simulink model "lab_4_equalizer_lms_buffer"  (R2012b)
settings: Solver=ode45  StartTime=0.0  StopTime=0.0012  RelTol=1e-3
values from neighbouring files (symbols this model uses):
  mu = 0.1    [lab_4_parameters.m]
  Ts = 1/Rs    (= 2.23214285714e-06)    [lab_4_parameters.m]
undefined symbols (not defined in the file or in its folder): dfilt, Fs, sided, Two
libraries: dspobslib x10, dspsigops x4, commsink2 x3, dspsnks4 x2, commchan3 x2, commdigbbndpm3 x2, dsparch4 x1, commrandsrc2 x1
settings Model: Creator=yuw  LastModifiedBy=yuw
settings OptimizationCC: InlineInvariantSignals=on  InitFltsAndDblsToZero=on
settings DebuggingCC: SaveWithParameterizedLinksMsg=none  SignalResolutionControl=TryResolveAllWithWarning  MultiTaskDSMMsg=warning  MultiTaskCondExecSysMsg=none  StrictBusMsg=None
settings RTWCC: IncludeERTFirstTime=on
settings GRTTargetCC: TargetFcnLib=ansi_tfl_tmw.mat  CombineOutputUpdateFcns=off  GRTInterface=on

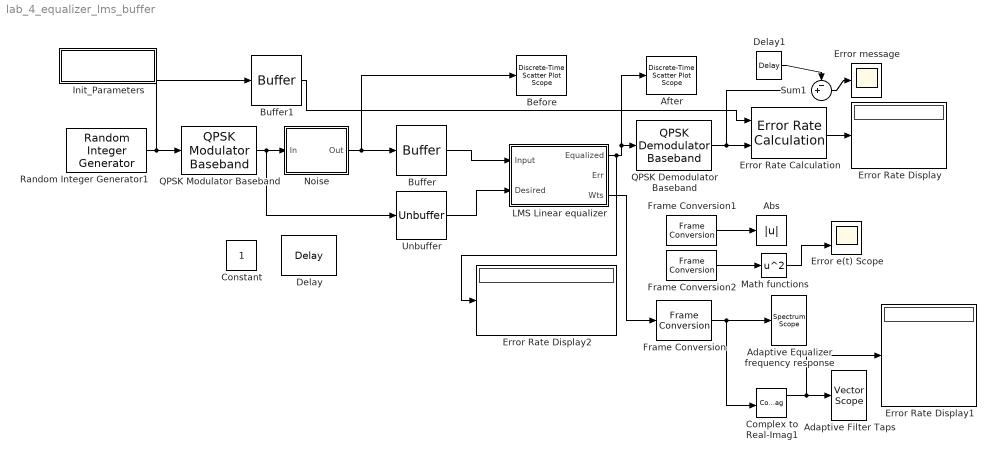
== system lab_4_equalizer_lms_buffer ==
  Abs : Abs
  Adaptive Equalizer frequency response : dspsnks4/Spectrum Scope  ScopeProperties=on  Domain=Frequency  HorizSpan=1  UseBuffer=off  BufferSize=128  Overlap=64  TreatMby1Signals=One channel  inpFftLenInherit=on  FFTlength=128  numAvg=2  DisplayProperties=off  AxisGrid=on  Memory=off  FrameNumber=on  AxisLegend=off  AxisZoom=off  OpenScopeAtSimStart=on  OpenScopeImmediately=off  FigPos=[8 424 450 170]  AxisProperties=off  XUnits=Hertz  XRange=Two-sided ((-Fs/2...Fs/2])  XDisplay=0  InheritXIncr=off  XIncr=1e-5  XLabel=Samples  XLimit=Auto  YUnits=dBW/Hertz  XMax=1  XMin=0  YLabel=Magnitude-squared, dB  LineProperties=off  LineStyles=--  LineMarkers=None  LineColors=[1 0 0]  wintypeSpecScope=Hann  RsSpecScope=50  betaSpecScope=5  winsampSpecScope=Periodic  XAxisParamsVer=6.8  isFrameUpgraded=on
      link override Periodogram: inheritFFT=off  inheritTs=off
      settings: YMin=-5.7892131592501  YMax=-3.17780882405879
  Adaptive Filter Taps : dspsnks4/Vector Scope  ScopeProperties=on  Domain=User-defined  HorizSpan=1  DisplayProperties=off  AxisGrid=on  Memory=off  FrameNumber=on  AxisLegend=off  AxisZoom=off  OpenScopeAtSimStart=on  OpenScopeImmediately=off  FigPos=[486 427 450 170]  AxisProperties=off  XUnits=Hertz  XRange=[0...Fs/2]  InheritXIncr=off  XIncr=1  XLabel=Coefficient Index  XLimit=Auto  XMin=0  XMax=1  XStart=0  YUnits=dB  YLabel=Amplitude  LineProperties=off  LineMarkers=.  XAxisParamsVer=6.8
      settings: YMin=-0.176505999051535  YMax=1.03663535601714
  After : commsink2/Discrete-Time Scatter Plot Scope  Tag=ScatterPlot  sampPerSymb=1  offsetEye=0  numTraces=400  numNewFrames=10  LineMarkers=.  LineColors=b  fading=on  render=on  AxisGrid=on  xMin=-1.5  xMax=1.5  yMin=-1.5  yMax=1.5  inphaseLabel=In-phase Amplitude  quadratureLabel=Quadrature Amplitude  openScopeAtSimStart=off  FrameNumber=off  FigPos=[420 374 400 400]  figTitle=Scatter Plot  numLinesMax=8  block_type_=scatter
  Before : commsink2/Discrete-Time Scatter Plot Scope  Tag=ScatterPlot  sampPerSymb=1  offsetEye=0  numTraces=400  numNewFrames=10  LineMarkers=.  LineColors=b  fading=on  render=on  AxisGrid=on  xMin=-1.5  xMax=1.5  yMin=-1.5  yMax=1.5  inphaseLabel=In-phase Amplitude  quadratureLabel=Quadrature Amplitude  openScopeAtSimStart=off  FrameNumber=off  FigPos=[10 374 400 400]  figTitle=Scatter Plot  numLinesMax=8  block_type_=scatter
  Buffer : Buffer  N=4
  Buffer1 : Buffer  N=10
  Complex to Real-Imag1 : ComplexToRealImag
  Constant : Constant
  Delay : dspsigops/Delay  InputProcessing=Inherited (this choice will be removed - see release notes)  dly_unit=Samples  delay=0  ic_detail=off  dif_ic_for_ch=off  dif_ic_for_dly=off  ic=0  reset_popup=None
  Delay1 : dspsigops/Delay  InputProcessing=Inherited (this choice will be removed - see release notes)  dly_unit=Samples  delay=4  ic_detail=off  dif_ic_for_ch=off  dif_ic_for_dly=off  ic=0  reset_popup=None
  Error Rate Calculation : commsink2/Error Rate Calculation  N=4  st_delay=0  cp_mode=Entire frame  subframe=[]  PMode=Port  WsName=ErrorVec  RsMode2=off  stop=off  numErr=100  maxBits=1e6
  Error Rate Display : Display
  Error Rate Display1 : Display
  Error Rate Display2 : Display
  Error e(t) Scope : Scope  NumInputPorts=2
      settings: TimeRange=1  YMin=5.55112e-017~-5  YMax=1.1~5  MaxDataPoints=10000
  Error message : Scope
      settings: TimeRange=1  YMin=-3  YMax=0  MaxDataPoints=10000
  Frame Conversion : FrameConversion
  Frame Conversion1 : FrameConversion  OutFrame=Sample-based
  Frame Conversion2 : FrameConversion  OutFrame=Sample-based
  Init_Parameters : Subsystem
      settings: OpenFcn=lab_4_parameters
      mask Display: disp('lab_4_parameters')
  LMS Linear equalizer : Subsystem
  Math functions : Math  Operator=square  SaturateOnIntegerOverflow=on
  Noise : Subsystem
  QPSK Demodulator Baseband : commdigbbndpm3/QPSK Demodulator Baseband  Ph=pi/4  Dec=Gray  OutType=Integer  DecType=Hard decision  VarSource=Dialog  Variance=1  outDtype1=Inherit via internal rule  outDtype2=Inherit via internal rule  derotateFactorWordLen=16
  QPSK Modulator Baseband : commdigbbndpm3/QPSK Modulator Baseband  InType=Integer  Enc=Gray  Ph=pi/4  outDtype=double  outWordLen=16  outUDDataType=sfix(16)  outFracLenMode=Best precision  outFracLen=15
  Random Integer Generator1 : commrandsrc2/Random Integer Generator  mul=4  seed=12345  Ts=Ts  frameBased=on  sampPerFrame=100  orient=off  outDataType=double
  Sum1 : Sum  Inputs=-+|  SaturateOnIntegerOverflow=on  InputSameDT=on  OutDataTypeStr=Inherit: Same as first input
  Unbuffer : Unbuffer
  wires:
  Noise/1(Out) -> Before/1, Buffer/1
  QPSK Modulator Baseband/1 -> Noise/1(In), Unbuffer/1
  Random Integer Generator1/1 -> QPSK Modulator Baseband/1, Buffer1/1
  QPSK Demodulator Baseband/1 -> Error Rate Calculation/2
  Error Rate Calculation/1 -> Error Rate Display/1
  Frame Conversion/1 -> Adaptive Equalizer frequency response/1, Complex to Real-Imag1/1
  Complex to Real-Imag1/1 -> Adaptive Filter Taps/1, Error Rate Display1/1
  Frame Conversion1/1 -> Abs/1
  Frame Conversion2/1 -> Math functions/1
  Math functions/1 -> Error e(t) Scope/2
  Sum1/1 -> Error message/1
  Delay1/1 -> Sum1/1
  LMS Linear equalizer/1(Equalized) -> After/1, QPSK Demodulator Baseband/1, Error Rate Display2/1
  LMS Linear equalizer/3(Wts) -> Frame Conversion/1
  Unbuffer/1 -> LMS Linear equalizer/2(Desired)
  Buffer1/1 -> Error Rate Calculation/1
  Buffer/1 -> LMS Linear equalizer/1(Input)

== system lab_4_equalizer_lms_buffer/Init_Parameters ==

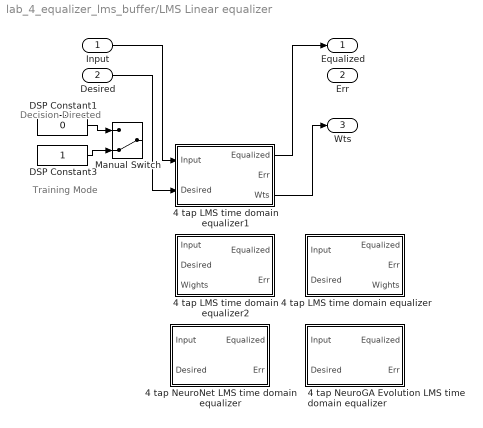
== system lab_4_equalizer_lms_buffer/LMS Linear equalizer ==
  note: Decision Directed
  note: Training Mode
  Input : Inport
  Desired : Inport  Port=2
  4 tap LMS time domain equalizer : Subsystem
  4 tap LMS time domain equalizer1 : Subsystem
  4 tap LMS time domain equalizer2 : Subsystem
  4 tap NeuroGA Evolution LMS time domain equalizer : Subsystem
  4 tap NeuroNet LMS time domain equalizer : Subsystem
  DSP Constant1 : Constant  Value=0  VectorParams1D=off  FramePeriod=1
      settings: SamplingMode=Frame based
  DSP Constant3 : Constant  VectorParams1D=off  FramePeriod=1
      settings: SamplingMode=Frame based
  Manual Switch : ManualSwitch  CurrentSetting=0
  Equalized : Outport
  Err : Outport  Port=2
  Wts : Outport  Port=3
  wires:
  DSP Constant3/1 -> Manual Switch/2
  DSP Constant1/1 -> Manual Switch/1
  Input/1 -> 4 tap LMS time domain equalizer1/1(Input)
  Desired/1 -> 4 tap LMS time domain equalizer1/2(Desired)
  4 tap LMS time domain equalizer1/1(Equalized) -> Equalized/1
  4 tap LMS time domain equalizer1/3(Wts) -> Wts/1

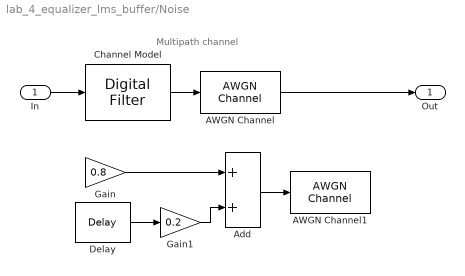
== system lab_4_equalizer_lms_buffer/Noise ==
  note: Multipath channel
  In : Inport
  AWGN Channel : commchan3/AWGN Channel  InputProcessing=Inherited (this choice will be removed - see release notes)  seed=67  noiseMode="Signal to noise ratio  (SNR)"  EbNodB=EbNodB  EsNodB=10  SNRdB=40  bitsPerSym=1  Ps=1  Tsym=Ts  variance=1
  AWGN Channel1 : commchan3/AWGN Channel  InputProcessing=Inherited (this choice will be removed - see release notes)  seed=67  noiseMode="Signal to noise ratio  (SNR)"  EbNodB=EbNodB  EsNodB=10  SNRdB=40  bitsPerSym=1  Ps=1  Tsym=Ts  variance=1
  Add : Sum
  Channel Model : dsparch4/Digital Filter  TypePopup=FIR (all zeros)  IIRFiltStruct=Direct form I transposed  AllPoleFiltStruct=Direct form transposed  FIRFiltStruct=Direct form transposed  CoeffSource=Specify via dialog  NumCoeffs=[1 -.3 .1 .2j]  DenCoeffs=[1 0.1]  BiQuadCoeffs=[1 0.3 0.4 1 0.1 0.2]  LatticeCoeffs=[0.2 0.4]  denIgnore=on  FiltPerSampPopup=One filter per frame  IC=0  ICnum=0  ICden=0  roundingMode=Floor  overflowMode=off  ScaleValues=1  scaleValueFracLength=14  stageInFracLength=15  stageOutFracLength=15  FilterSource=Specify via dialog  dfiltObjectName=dfilt.dffir([1 2 1])  InputProcessing=Inherited (this choice will be removed - see release notes)
  Delay : dspsigops/Delay  InputProcessing=Inherited (this choice will be removed - see release notes)  dly_unit=Samples  delay=1  ic_detail=off  dif_ic_for_ch=off  dif_ic_for_dly=off  ic=0  reset_popup=None
  Gain : Gain  Gain=0.8
  Gain1 : Gain  Gain=0.2
  Out : Outport
  wires:
  Gain1/1 -> Add/2
  Delay/1 -> Gain1/1
  Gain/1 -> Add/1
  Add/1 -> AWGN Channel1/1
  Channel Model/1 -> AWGN Channel/1
  In/1 -> Channel Model/1
  AWGN Channel/1 -> Out/1

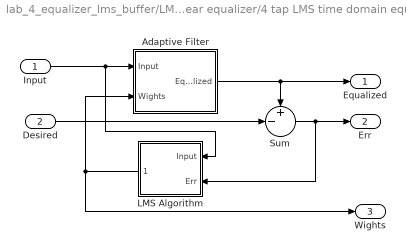
== system lab_4_equalizer_lms_buffer/LMS Linear equalizer/4 tap LMS time domain equalizer ==
  Input : Inport
  Desired : Inport  Port=2
  Adaptive Filter : Subsystem
  LMS Algorithm : Subsystem
  Sum : Sum  Inputs=+-|
  Equalized : Outport
  Err : Outport  Port=2
  Wights : Outport  Port=3
  wires:
  Desired/1 -> Sum/2
  LMS Algorithm/1(Wights) -> Wights/1, Adaptive Filter/2(Wights)
  Input/1 -> LMS Algorithm/1(Input), Adaptive Filter/1(Input)
  Sum/1 -> LMS Algorithm/2(Err), Err/1
  Adaptive Filter/1(Equalized) -> Sum/1, Equalized/1

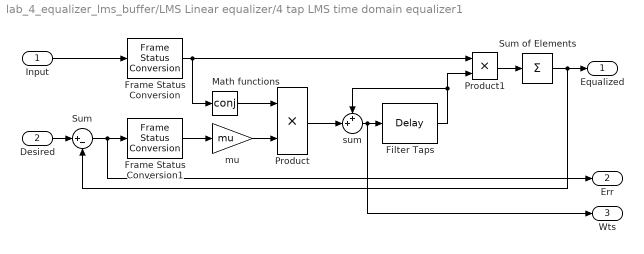
== system lab_4_equalizer_lms_buffer/LMS Linear equalizer/4 tap LMS time domain equalizer1 ==
  Input : Inport
  Desired : Inport  Port=2
  Filter Taps : dspsigops/Delay  InputProcessing=Inherited (this choice will be removed - see release notes)  dly_unit=Samples  delay=4  ic_detail=on  dif_ic_for_ch=off  dif_ic_for_dly=off  ic=0  reset_popup=None
  Frame Status Conversion : dspobslib/Frame Status Conversion  growRefPort=off  outframe=Sample-based
  Frame Status Conversion1 : dspobslib/Frame Status Conversion  growRefPort=off  outframe=Sample-based
  Math functions : Math  Operator=conj  SaturateOnIntegerOverflow=on
  Product : Product  SaturateOnIntegerOverflow=on
  Product1 : Product  SaturateOnIntegerOverflow=on
  Sum : Sum  Inputs=|+-
  Sum of Elements : Sum  Inputs=+
  mu : Gain  Gain=mu  SaturateOnIntegerOverflow=on  OutDataTypeStr=Inherit: Same as input  ParamDataTypeStr=Inherit: Same as input
  sum : Sum  Inputs=++|  SaturateOnIntegerOverflow=on  InputSameDT=on  OutDataTypeStr=Inherit: Same as first input
  Equalized : Outport
  Err : Outport  Port=2
  Wts : Outport  Port=3
  wires:
  Input/1 -> Frame Status Conversion/1
  Sum/1 -> Frame Status Conversion1/1, Err/1
  Desired/1 -> Sum/1
  Math functions/1 -> Product/1
  Frame Status Conversion/1 -> Math functions/1, Product1/1
  Product1/1 -> Sum of Elements/1
  Sum of Elements/1 -> Equalized/1, Sum/2
  Product/1 -> sum/2
  sum/1 -> Filter Taps/1, Wts/1
  Filter Taps/1 -> Product1/2, sum/1
  mu/1 -> Product/2
  Frame Status Conversion1/1 -> mu/1

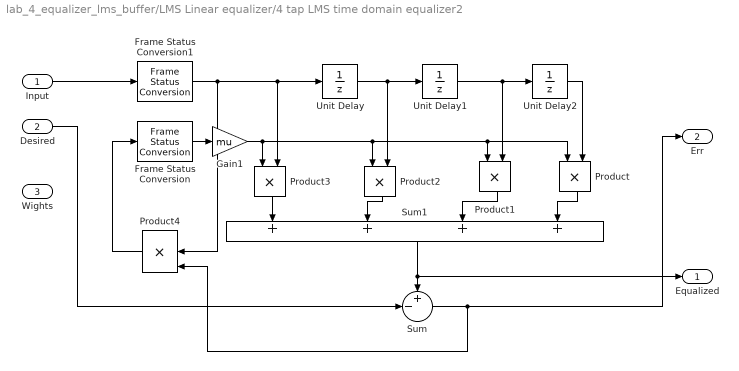
== system lab_4_equalizer_lms_buffer/LMS Linear equalizer/4 tap LMS time domain equalizer2 ==
  Input : Inport
  Desired : Inport  Port=2
  Wights : Inport  Port=3
  Frame Status Conversion : dspobslib/Frame Status Conversion  growRefPort=off  outframe=Sample-based
  Frame Status Conversion1 : dspobslib/Frame Status Conversion  growRefPort=off  outframe=Sample-based
  Gain1 : Gain  Gain=mu
  Product{,1..3} (4 alike) : Product  RndMeth=Zero
  Product4 : Product  Inputs=3  RndMeth=Zero
  Sum : Sum  Inputs=+-|
  Sum1 : Sum  Inputs=++++
  Unit Delay : UnitDelay
  Unit Delay1 : UnitDelay
  Unit Delay2 : UnitDelay
  Equalized : Outport
  Err : Outport  Port=2
  wires:
  Product4/1 -> Frame Status Conversion/1
  Frame Status Conversion1/1 -> Product4/2, Product3/2, Unit Delay/1
  Input/1 -> Frame Status Conversion1/1
  Frame Status Conversion/1 -> Gain1/1
  Sum/1 -> Product4/3, Err/1
  Gain1/1 -> Product/1, Product1/1, Product2/1, Product3/1
  Desired/1 -> Sum/2
  Sum1/1 -> Sum/1, Equalized/1
  Product/1 -> Sum1/4
  Product1/1 -> Sum1/3
  Product2/1 -> Sum1/2
  Product3/1 -> Sum1/1
  Unit Delay2/1 -> Product/2
  Unit Delay1/1 -> Product1/2, Unit Delay2/1
  Unit Delay/1 -> Product2/2, Unit Delay1/1

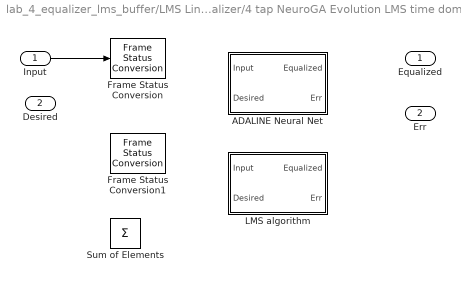
== system lab_4_equalizer_lms_buffer/LMS Linear equalizer/4 tap NeuroGA Evolution LMS time domain equalizer ==
  Input : Inport
  Desired : Inport  Port=2
  ADALINE Neural Net : Subsystem
  Frame Status Conversion : dspobslib/Frame Status Conversion  growRefPort=off  outframe=Sample-based
  Frame Status Conversion1 : dspobslib/Frame Status Conversion  growRefPort=off  outframe=Sample-based
  LMS algorithm : Subsystem
  Sum of Elements : Sum  Inputs=+
  Equalized : Outport
  Err : Outport  Port=2
  wires:
  Input/1 -> Frame Status Conversion/1

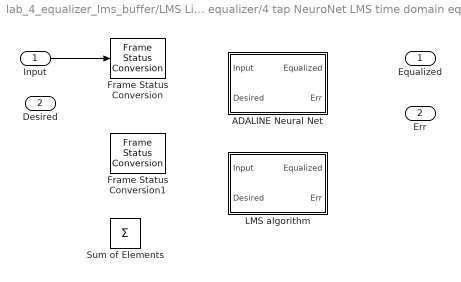
== system lab_4_equalizer_lms_buffer/LMS Linear equalizer/4 tap NeuroNet LMS time domain equalizer ==
  Input : Inport
  Desired : Inport  Port=2
  ADALINE Neural Net : Subsystem
  Frame Status Conversion : dspobslib/Frame Status Conversion  growRefPort=off  outframe=Sample-based
  Frame Status Conversion1 : dspobslib/Frame Status Conversion  growRefPort=off  outframe=Sample-based
  LMS algorithm : Subsystem
  Sum of Elements : Sum  Inputs=+
  Equalized : Outport
  Err : Outport  Port=2
  wires:
  Input/1 -> Frame Status Conversion/1

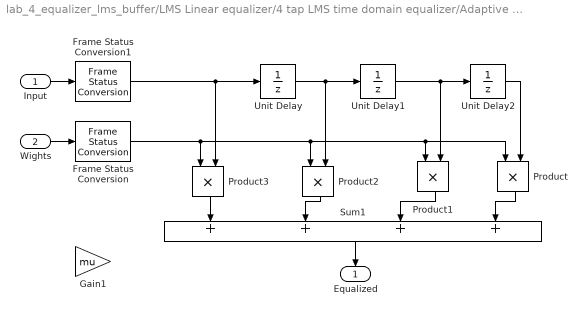
== system lab_4_equalizer_lms_buffer/LMS Linear equalizer/4 tap LMS time domain equalizer/Adaptive Filter ==
  Input : Inport
  Wights : Inport  Port=2
  Frame Status Conversion : dspobslib/Frame Status Conversion  growRefPort=off  outframe=Sample-based
  Frame Status Conversion1 : dspobslib/Frame Status Conversion  growRefPort=off  outframe=Sample-based
  Gain1 : Gain  Gain=mu
  Product{,1..3} (4 alike) : Product  RndMeth=Zero
  Sum1 : Sum  Inputs=++++
  Unit Delay : UnitDelay
  Unit Delay1 : UnitDelay
  Unit Delay2 : UnitDelay
  Equalized : Outport
  wires:
  Sum1/1 -> Equalized/1
  Wights/1 -> Frame Status Conversion/1
  Input/1 -> Frame Status Conversion1/1
  Frame Status Conversion1/1 -> Product3/2, Unit Delay/1
  Frame Status Conversion/1 -> Product/1, Product1/1, Product2/1, Product3/1
  Product/1 -> Sum1/4
  Product1/1 -> Sum1/3
  Product2/1 -> Sum1/2
  Product3/1 -> Sum1/1
  Unit Delay2/1 -> Product/2
  Unit Delay1/1 -> Product1/2, Unit Delay2/1
  Unit Delay/1 -> Product2/2, Unit Delay1/1

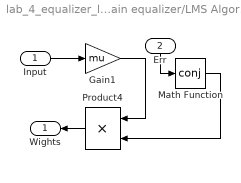
== system lab_4_equalizer_lms_buffer/LMS Linear equalizer/4 tap LMS time domain equalizer/LMS Algorithm ==
  Input : Inport
  Err : Inport  Port=2
  Gain1 : Gain  Gain=mu
  Math Function : Math  Operator=conj  SaturateOnIntegerOverflow=on
  Product4 : Product  RndMeth=Zero
  Wights : Outport
  wires:
  Product4/1 -> Wights/1
  Err/1 -> Math Function/1
  Input/1 -> Gain1/1
  Math Function/1 -> Product4/2
  Gain1/1 -> Product4/1

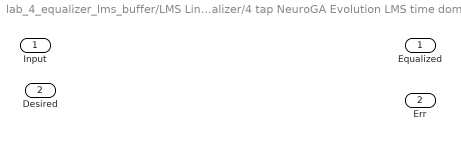
== system lab_4_equalizer_lms_buffer/LMS Linear equalizer/4 tap NeuroGA Evolution LMS time domain equalizer/ADALINE Neural Net ==
  Input : Inport
  Desired : Inport  Port=2
  Equalized : Outport
  Err : Outport  Port=2

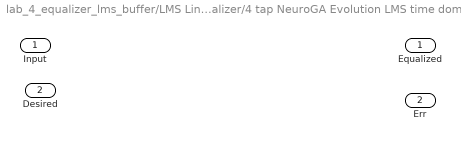
== system lab_4_equalizer_lms_buffer/LMS Linear equalizer/4 tap NeuroGA Evolution LMS time domain equalizer/LMS algorithm ==
  Input : Inport
  Desired : Inport  Port=2
  Equalized : Outport
  Err : Outport  Port=2

== system lab_4_equalizer_lms_buffer/LMS Linear equalizer/4 tap NeuroNet LMS time domain equalizer/ADALINE Neural Net ==
  Input : Inport
  Desired : Inport  Port=2
  Equalized : Outport
  Err : Outport  Port=2

== system lab_4_equalizer_lms_buffer/LMS Linear equalizer/4 tap NeuroNet LMS time domain equalizer/LMS algorithm ==
  Input : Inport
  Desired : Inport  Port=2
  Equalized : Outport
  Err : Outport  Port=2
